simulink model "Publish_Subscribe_Model_Test"  (R2017a)
settings: Solver=VariableStepAuto  StartTime=0.0  StopTime=inf  RelTol=1e-3
undefined symbols (not defined in the file): Angular, Linear
libraries: robotlib x3
settings Model: Creator=francesco  LastModifiedBy=francesco

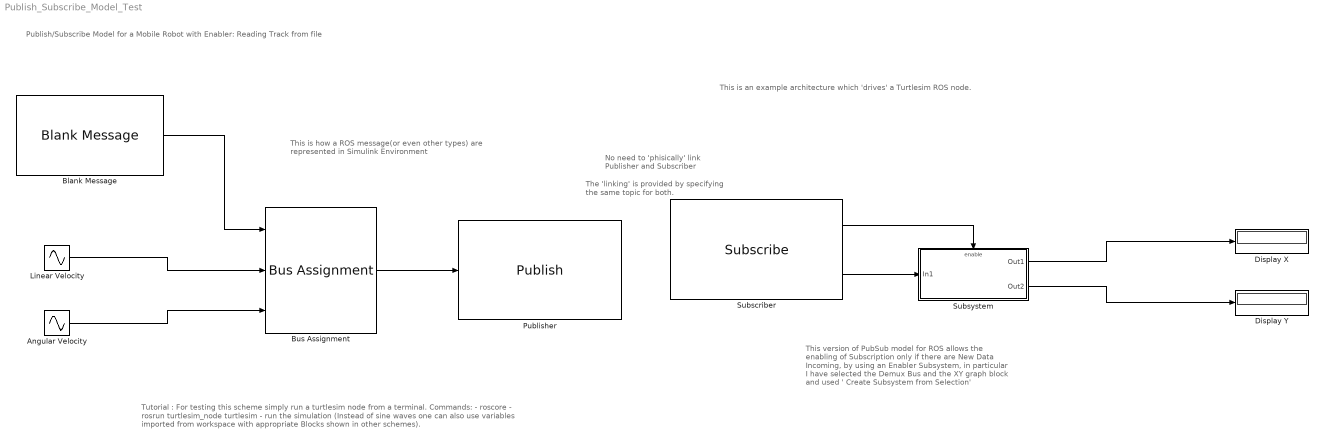
== system Publish_Subscribe_Model_Test ==
  note: Tutorial : For testing this scheme simply run a turtlesim node from a terminal.
      | Commands:
      | - roscore
      | - rosrun turtlesim_node turtlesim
      | - run the simulation (Instead of sine waves one can also use variables imported from workspace with appropriate Blocks shown in other schemes).
  note: This is an example architecture which 'drives' a Turtlesim ROS node.
  note: This is how a ROS message(or even other types)
      |  are represented in Simulink Environment
  note: This version of PubSub model for ROS allows
      | the enabling of Subscription only if there are New
      | Data Incoming, by using an Enabler Subsystem, in
      | particular I have selected the Demux Bus and the
      | XY graph block and used ' Create Subsystem from
      | Selection'
  note: Publish/Subscribe Model for a Mobile Robot with Enabler: Reading Track from file
  note: The 'linking' is provided by specifying
      | the same topic for both.
  note: No need to 'phisically' link
      | Publisher and Subscriber
  Angular Velocity : Sin  SampleTime=0
  Blank Message : robotlib/Blank Message  SourceLibraryInfo=This block requires Robotics System Toolbox  messageType=geometry_msgs/Twist  SampleTime=inf
      settings: SourceProductBaseCode=RO
  Bus Assignment : BusAssignment  AssignedSignals=Linear.X,Angular.Z
  Display X : Display
  Display Y : Display
  Linear Velocity : Sin  SampleTime=0
  Publisher : robotlib/Publish  SourceLibraryInfo=This block requires Robotics System Toolbox  topicSource=Select from ROS network  topic=/turtle1/cmd_vel  messageType=geometry_msgs/Twist  messageQueueLength=1
      settings: SourceProductBaseCode=RO
  Subscriber : robotlib/Subscribe  SourceLibraryInfo=This block requires Robotics System Toolbox  topicSource=Select from ROS network  topic=/turtle1/pose  messageType=turtlesim/Pose  sampleTime=-1  messageQueueLength=1
      settings: SourceProductBaseCode=RO
  Subsystem : Subsystem
  wires:
  Subscriber/2 -> Subsystem/1(In1)
  Blank Message/1 -> Bus Assignment/1
  Bus Assignment/1 -> Publisher/1
  Subsystem/1(Out1) -> Display X/1
  Subsystem/2(Out2) -> Display Y/1
  Subscriber/1 -> Subsystem/Enable
  Linear Velocity/1 -> Bus Assignment/2
  Angular Velocity/1 -> Bus Assignment/3

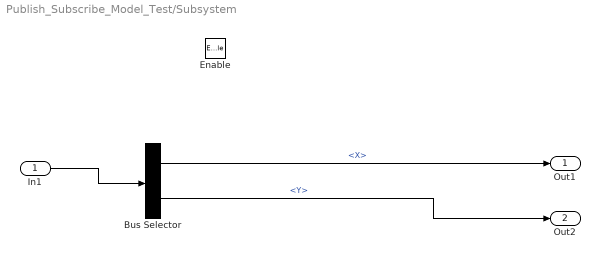
== system Publish_Subscribe_Model_Test/Subsystem ==
  In1 : Inport
  Enable : EnablePort
  Bus Selector : BusSelector  OutputSignals=X,Y
  Out1 : Outport
  Out2 : Outport  Port=2
  wires:
  In1/1 -> Bus Selector/1
  Bus Selector/2 -> Out2/1  "<Y>"
  Bus Selector/1 -> Out1/1  "<X>"
